simulink model "WiperCtrl"  (R2023b)
settings: Solver=FixedStepDiscrete  StartTime=0.0  StopTime=4  FixedStep=5e-5  RelTol=1e-3  EnableMultiTasking=on
values from neighbouring files (symbols this model uses):
  MC_Hardware_Motor_Mechinal_Fric = 0    [ModelParamSet.m]
  MC_Hardware_Motor_Mechinal_Inertia = 1.03e-2    (= 0.0103)    [ModelParamSet.m]
  MC_Hardware_Motor_Mechinal_TF = 8.59e-2    (= 0.0859)    [ModelParamSet.m]
  MC_Hardware_Motor_Rotor_BEMFCoff = 4.294    [ModelParamSet.m]
  MC_Hardware_Motor_Rotor_Pn = 4    [ModelParamSet.m]
  MC_Hardware_Motor_Stator_Ld = 5.6345e-5    (= 5.6345e-05)    [ModelParamSet.m]
  MC_Hardware_Motor_Stator_Lq = 5.6345e-5    (= 5.6345e-05)    [ModelParamSet.m]
  MC_Hardware_Motor_Stator_Rs = 2.86e-2    (= 0.0286)    [ModelParamSet.m]
  MC_Hardware_Power_DC = 13.5    [ModelParamSet.m]
  MC_Hardware_Sample_CurrentNoise = 1e-15    [ModelParamSet.m]
  MC_Hardware_Sample_Rs = 1e-3    (= 0.001)    [ModelParamSet.m]
  MC_Hardware_Sample_VbusNoise = 1e-15    [ModelParamSet.m]
  MC_Sim_BaseStep = 5e-8    (= 5e-08)    [ModelParamSet.m]
  MC_Sim_HighFrequenceStep = 5e-5    (= 5e-05)    [ModelParamSet.m]
  MC_SVPWM_DutyMax = 0.98    [ModelParamSet.m]
  MC_SVPWM_DutyMin = 0.02    [ModelParamSet.m]
libraries: simulink x12, spsVoltageMeasurementLib x2, spsDCVoltageSourceLib x1, spsGroundLib x1, spsPermanentMagnetSynchronousMachineLib x1, spsSeriesRLCBranchLib x1, spsThreePhaseVIMeasurementLib x1, spsUniversalBridgeLib x1, spspowerguiLib x1
(part 1 of 2)
settings Model: SimulationMode=accelerator  Creator=YXuan  LastModifiedBy=YXuan
settings SolverCC: AllowMultiTaskInputOutput=on  PositivePriorityOrder=on  AutoInsertRateTranBlk=on
settings OptimizationCC: DefaultParameterBehavior=Inlined  EnhancedBackFolding=on  PassReuseOutputArgsAs=Individual arguments  ZeroExternalMemoryAtStartup=off  ZeroInternalMemoryAtStartup=off  OptimizeBlockOrder=speed  DifferentSizesBufferReuse=on  OptimizationCustomize=off  EfficientTunableParamExpr=on
settings DebuggingCC: ParameterPrecisionLossMsg=none  ParameterTunabilityLossMsg=error
settings SFSimCC: MATLABDynamicMemAlloc=off
settings RTWCC: Description=Embedded Coder  SystemTargetFile=ert.tlc  GenCodeOnly=on  TemplateMakefile=ert_default_tmf  Toolchain=Microsoft Visual C++ 2022 v17.0 | nmake (64-bit Windows)
settings CodeAppCC: ForceParamTrailComments=on  IgnoreCustomStorageClasses=off  OperatorAnnotations=on  SimulinkDataObjDesc=on  SFDataObjDesc=on  InsertBlockDesc=on
settings ERTTargetCC: TargetLangStandard=C99 (ISO)  GenerateSampleERTMain=on  InlinedParameterPlacement=NonHierarchical  ERTCustomFileTemplate=example_file_process.tlc

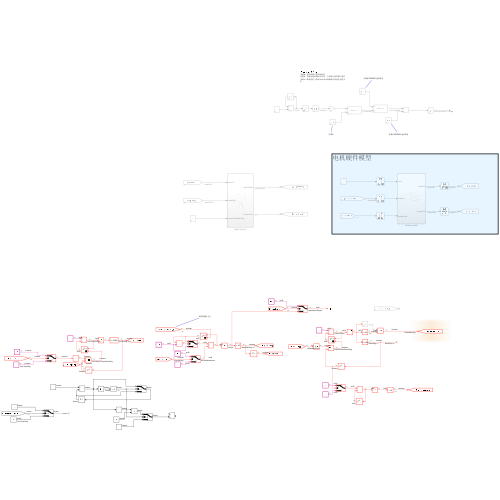
[thumbnail: Simulink's stored preview of the top-level diagram]
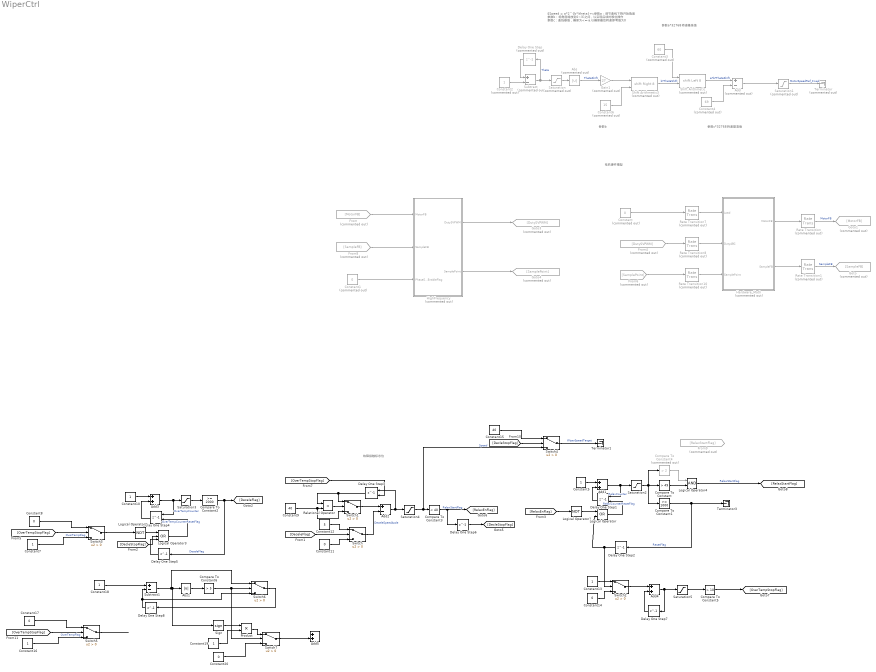
== system WiperCtrl ==
  note: 故障接触标志位
  note: $Speed = a*2^{b*\theta}+c$
      | 参数a：调节曲线下降开始角度
      | 参数b：将角度缩放到0~31之间，以实现后续的移位操作
      | 参数c：曲线基值，确保为<=-a,以确保最后转速参考值为0
  note: 参数a*32768/转速基准值
  note: 电机硬件模型
  note: 参数c*32768/转速基准值
  note: 参数b
  Abs : Abs  Commented=on  SaturateOnIntegerOverflow=off
  Abs1 : Abs  SaturateOnIntegerOverflow=off
  Add : Sum  Commented=on  Inputs=+-
  Add{1,3..5} (4 alike) : Sum
  Add2 : Sum  Inputs=+-
  Compare To Constant : simulink/Logic and Bit Operations/Compare To Constant  relop=>  const=49  OutDataTypeStr=boolean
  Compare To Constant1 : simulink/Logic and Bit Operations/Compare To Constant  relop=>=  const=1000  OutDataTypeStr=boolean
  Compare To Constant2 : simulink/Logic and Bit Operations/Compare To Constant  relop=>=  const=2000  OutDataTypeStr=boolean
  Compare To Constant3 : simulink/Logic and Bit Operations/Compare To Constant  relop=<  const=40  OutDataTypeStr=boolean
  Compare To Constant4 : simulink/Logic and Bit Operations/Compare To Constant  Commented=on  relop=>  const=2  OutDataTypeStr=boolean
  Compare To Constant5 : simulink/Logic and Bit Operations/Compare To Constant  relop=>  const=10  OutDataTypeStr=boolean
  Compare To Constant6 : simulink/Logic and Bit Operations/Compare To Constant  relop=>  const=5  OutDataTypeStr=boolean
  Constant : Constant  Commented=on  Value=0
  Constant1 : Constant  Commented=on  Value=0  OutDataTypeStr=boolean
  Constant{5,10,13,18..19} (5 alike) : Constant  OutDataTypeStr=int32
  Constant11 : Constant  Value=0  OutDataTypeStr=int32
  Constant12 : Constant  Value=5  OutDataTypeStr=int32
  Constant14 : Constant  Value=0  OutDataTypeStr=int32
  Constant15 : Constant  Value=40  OutDataTypeStr=int32
  Constant16 : Constant  OutDataTypeStr=boolean
  Constant17 : Constant  Value=0  OutDataTypeStr=boolean
  Constant2 : Constant  Commented=on  OutDataTypeStr=int32
  Constant20 : Constant  Value=0  OutDataTypeStr=int32
  Constant3 : Constant  Commented=on  Value=60  OutDataTypeStr=int32
  Constant4 : Constant  Commented=on  Value=69  OutDataTypeStr=int16
  Constant6 : Constant  Commented=on  Value=15  OutDataTypeStr=int16
  Constant7 : Constant  OutDataTypeStr=boolean
  Constant8 : Constant  Value=0  OutDataTypeStr=boolean
  Constant9 : Constant  Value=40  OutDataTypeStr=int32
  Delay One Step : Delay  Commented=on  DelayLength=1  InitialCondition=int32(32768)
  Delay One Step1 : Delay  DelayLength=1  InitialCondition=int32(0)  ExternalReset=Level
      settings: InputPortMap=u0,r5
  Delay One Step2 : Delay  DelayLength=1  InitialCondition=boolean(0)
  Delay One Step3 : Delay  DelayLength=1  InitialCondition=60  ExternalReset=Level
      settings: InputPortMap=u0,r5
  Delay One Step4 : Delay  DelayLength=1  InitialCondition=int32(0)  ExternalReset=Level
      settings: InputPortMap=u0,r5
  Delay One Step5 : Delay  DelayLength=1  InitialCondition=boolean(0)
  Delay One Step6 : Delay  DelayLength=1  InitialCondition=boolean(0)
  Delay One Step7 : Delay  DelayLength=1  InitialCondition=int32(0)
  Delay One Step8 : Delay  DelayLength=1
  From : From  Commented=on  GotoTag=MotorFB
  From4 : From  Commented=on  GotoTag=DutySVPWM
  From6 : From  Commented=on  GotoTag=SamplePoint
  From8 : From  Commented=on  GotoTag=SampleFB
  From9 : From  Commented=on  GotoTag=RelaxStartFlag
  Gain1 : Gain  Commented=on  Gain=27  ParamDataTypeStr=int16  OutDataTypeStr=int32  RndMeth=Simplest
  Goto : Goto  Commented=on  GotoTag=SampleFB
  Goto1 : Goto  Commented=on  GotoTag=MotorFB
  Goto3 : Goto  Commented=on  GotoTag=DutySVPWM
  Goto4 : Goto  Commented=on  GotoTag=SamplePoint
  Hardware_Math : Subsystem  Commented=on  SystemSampleTime=MC_Sim_BaseStep  VariantControl=MC_Hardware_Motor_Model ==1&MC_Hardware_MotorMOS_Model==1
  HighFrequency : Subsystem  Commented=on
  Logical Operator : Logic  Operator=OR  AllPortsSameDT=off  OutDataTypeStr=boolean
  Logical Operator1 : Logic  Operator=NOT  AllPortsSameDT=off  OutDataTypeStr=boolean
  Logical Operator2 : Logic  Operator=NOT  AllPortsSameDT=off  OutDataTypeStr=boolean
  Logical Operator3 : Logic  Operator=OR  Inputs=3  AllPortsSameDT=off  OutDataTypeStr=boolean
  Logical Operator4 : Logic  AllPortsSameDT=off  OutDataTypeStr=boolean
  Product : Product
  Rate Transition : RateTransition  Commented=on  OutPortSampleTime=MC_Sim_HighFrequenceStep
  Rate Transition1 : RateTransition  Commented=on  OutPortSampleTime=MC_Sim_HighFrequenceStep
  Rate Transition10 : RateTransition  Commented=on  OutPortSampleTime=MC_Sim_BaseStep
  Rate Transition7 : RateTransition  Commented=on  OutPortSampleTime=MC_Sim_BaseStep
  Rate Transition8 : RateTransition  Commented=on  OutPortSampleTime=MC_Sim_BaseStep
  Relational Operator : RelationalOperator  Operator=<  OutDataTypeStr=boolean  RndMeth=Simplest  InputSameDT=off
  Saturation : Saturate  Commented=on  UpperLimit=32768  LowerLimit=-32768  OutDataTypeStr=int32  RndMeth=Simplest
  Saturation1 : Saturate  Commented=on  UpperLimit=4800  LowerLimit=0
  Saturation2 : Saturate  UpperLimit=1500  LowerLimit=-1
  Saturation3 : Saturate  UpperLimit=2001  LowerLimit=-1
  Saturation4 : Saturate  UpperLimit=60  LowerLimit=30  OutDataTypeStr=int32  RndMeth=Simplest
  Saturation5 : Saturate  UpperLimit=20  LowerLimit=-1
  Shift Arithmetic : ArithShift  Commented=on  BitShiftNumberSource=Input port  BitShiftNumber=8  BitShiftDirection=Left
      settings: InputPortMap=u0,p1
  Shift Arithmetic3 : ArithShift  Commented=on  BitShiftNumberSource=Input port  BitShiftNumber=8  BitShiftDirection=Right
      settings: InputPortMap=u0,p1
  Sign : Signum
  Subtract : Sum  Commented=on  Inputs=+-
  Subtract1 : Sum  Inputs=+-
  Switch{,1..7} (8 alike) : Switch  Criteria=u2 > Threshold  SaturateOnIntegerOverflow=off  InputSameDT=off
  Terminator : Terminator  Commented=on
  Terminator1 : Terminator
  Terminator3 : Terminator
  wires:
  Hardware_Math/2(SampleFB) -> Rate Transition1/1
  Rate Transition8/1 -> Hardware_Math/2(DutyABC)
  Hardware_Math/1(MotorFB) -> Rate Transition/1
  From6/1 -> Rate Transition10/1
  From4/1 -> Rate Transition8/1
  Rate Transition1/1 -> Goto/1  "SampleFB"
  Constant/1 -> Rate Transition7/1
  Rate Transition10/1 -> Hardware_Math/3(SamplePoint)
  Rate Transition7/1 -> Hardware_Math/1(Load)
  Rate Transition/1 -> Goto1/1  "MotorFB"
  From8/1 -> HighFrequency/2(SampleFB)
  From/1 -> HighFrequency/1(MotorFB)
  Constant1/1 -> HighFrequency/3(PhaseShortEnableFlag)
  HighFrequency/2(SamplePoint) -> Goto4/1
  HighFrequency/1(DutySVPWM) -> Goto3/1
  Subtract/1 -> Saturation/1, Delay One Step/1  "Theta"
  Delay One Step/1 -> Subtract/1
  Constant2/1 -> Subtract/2
  Saturation/1 -> Abs/1
  Abs/1 -> Gain1/1  "ThetaShift"
  Constant3/1 -> Shift Arithmetic/1
  Shift Arithmetic/1 -> Add/1  "a*b*ThetaShift"
  Constant4/1 -> Add/2
  Shift Arithmetic3/1 -> Shift Arithmetic/2  "b*ThetaShift"
  Gain1/1 -> Shift Arithmetic3/1
  Constant6/1 -> Shift Arithmetic3/2
  Add/1 -> Saturation1/1
  Saturation1/1 -> Terminator/1  "MotorSpeedRef_Fixed"
  Constant5/1 -> Add1/1
  Add1/1 -> Saturation2/1, Delay One Step1/1  "RelaxCounter"
  Delay One Step1/1 -> Add1/2
  Saturation2/1 -> Compare To Constant/1, Compare To Constant4/1, Compare To Constant1/1
  Logical Operator4/1 -> [RelaxStartFlag]  "RelaxStartFlag"
  Compare To Constant1/1 -> Terminator3/1, Delay One Step2/1  "ResetFlag"
  Delay One Step2/1 -> Logical Operator/2, Switch2/2
  Logical Operator/1 -> Delay One Step1/2  "RelaxCounterResetFlag"
  Logical Operator1/1 -> Logical Operator/1
  Constant10/1 -> Add3/1
  Add3/1 -> Saturation3/1, Delay One Step4/1  "OverTempCounter"
  Delay One Step4/1 -> Add3/2
  Switch3/1 -> Logical Operator2/1
  Saturation3/1 -> Compare To Constant2/1
  Compare To Constant2/1 -> [DeceleFlag], Delay One Step5/1  "DeceleFlag"
  Logical Operator2/1 -> Logical Operator3/1
  Logical Operator3/1 -> Delay One Step4/2  "OverTempCounterResetFlag"
  Delay One Step5/1 -> Logical Operator3/3
  [DeceleFlag] -> Switch/2
  Constant11/1 -> Switch/3
  Constant12/1 -> Switch/1
  Switch/1 -> Add2/2  "DeceleSpeedAccle"
  Switch1/1 -> Add2/1
  Delay One Step3/1 -> Switch1/1, Relational Operator/1
  Constant9/1 -> Relational Operator/2, Switch1/3
  Relational Operator/1 -> Switch1/2
  Add2/1 -> Saturation4/1, Delay One Step3/1
  Saturation4/1 -> Switch4/3, Compare To Constant3/1  "Speed"
  Compare To Constant3/1 -> [RelaxEnFlag], Delay One Step6/1  "RelaxStartFlag"
  Compare To Constant4/1 -> Logical Operator4/1
  Compare To Constant/1 -> Logical Operator4/2
  [DecleStopFlag] -> Logical Operator3/2
  Delay One Step6/1 -> [DecleStopFlag]
  [RelaxEnFlag] -> Logical Operator1/1
  Constant13/1 -> Switch2/1
  Constant14/1 -> Switch2/3
  Switch2/1 -> Add4/1
  Add4/1 -> Saturation5/1, Delay One Step7/1
  Delay One Step7/1 -> Add4/2
  Saturation5/1 -> Compare To Constant5/1
  Compare To Constant5/1 -> [OverTempStopFlag]
  [OverTempStopFlag] -> Switch3/2
  Constant7/1 -> Switch3/3  "OverTempFlag"
  Constant8/1 -> Switch3/1
  [OverTempStopFlag] -> Delay One Step3/2
  [DecleStopFlag] -> Switch4/2
  Constant15/1 -> Switch4/1
  Switch4/1 -> Terminator1/1  "WiperSpeedTarget"
  Constant17/1 -> Switch5/1
  Constant16/1 -> Switch5/3  "OverTempFlag"
  [OverTempStopFlag] -> Switch5/2
  Switch5/1 -> ?
  Constant18/1 -> Subtract1/1
  Subtract1/1 -> Switch6/1, Sign/1, Abs1/1
  Delay One Step8/1 -> Subtract1/2, Switch6/3
  Compare To Constant6/1 -> Switch7/2, Switch6/2
  Switch6/1 -> Delay One Step8/1
  Abs1/1 -> Compare To Constant6/1
  Sign/1 -> Product/1
  Constant19/1 -> Product/2
  Product/1 -> Switch7/1
  Constant20/1 -> Switch7/3
  Switch7/1 -> Add5/2

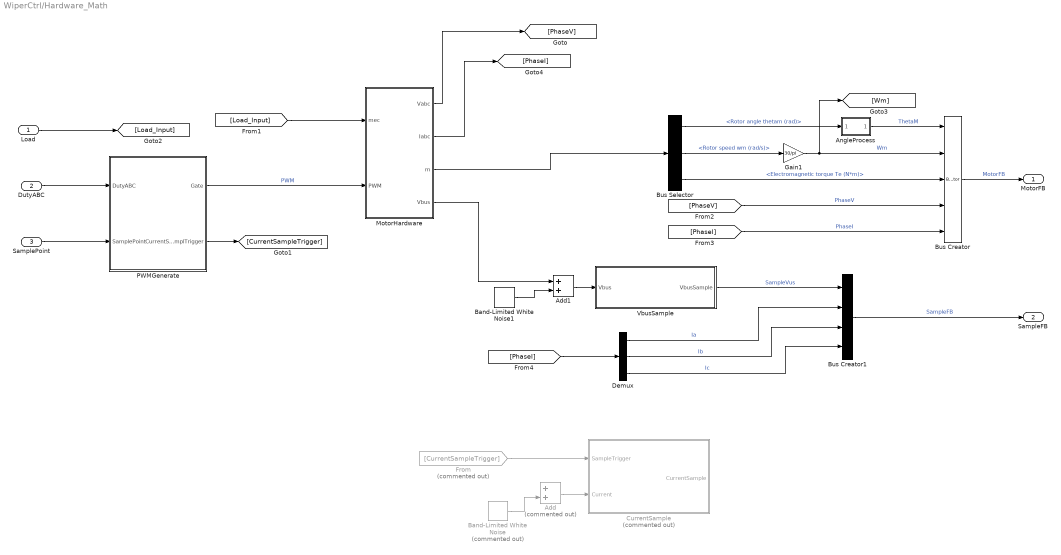
== system WiperCtrl/Hardware_Math ==
  Load : Inport
  DutyABC : Inport  Port=2
  SamplePoint : Inport  Port=3
  Add : Sum  Commented=on
  Add1 : Sum
  AngleProcess : Subsystem
  Band-Limited White Noise : simulink/Sources/Band-Limited White Noise  Commented=on  Cov=[MC_Hardware_Sample_CurrentNoise]  Ts=MC_Sim_BaseStep  seed=[23341]
  Band-Limited White Noise1 : simulink/Sources/Band-Limited White Noise  Cov=[MC_Hardware_Sample_VbusNoise]  Ts=MC_Sim_BaseStep  seed=[23341]
  Bus Creator : BusCreator  Inputs=5
  Bus Creator1 : BusCreator  Inputs=4
  Bus Selector : BusSelector  OutputSignals=Rotor angle thetam (rad),Rotor speed wm (rad/s),Electromagnetic torque Te (N*m)
  CurrentSample : Subsystem  Commented=on  Variant=on  VariantControlMode=label  VariantControl=CurrentSample  LabelModeActiveChoice=CurrentSample
  Demux : Demux  Outputs=3
  From : From  Commented=on  GotoTag=CurrentSampleTrigger
  Gain1 : Gain  Gain=30/pi
  MotorHardware : Subsystem
  PWMGenerate : Subsystem  SystemSampleTime=MC_Sim_BaseStep
  VbusSample : Subsystem
  MotorFB : Outport
  SampleFB : Outport  Port=2
  wires:
  Band-Limited White Noise/1 -> Add/2
  Add/1 -> CurrentSample/2(Current)
  Add1/1 -> VbusSample/1(Vbus)
  Band-Limited White Noise1/1 -> Add1/2
  From/1 -> CurrentSample/1(SampleTrigger)
  PWMGenerate/2(CurrentSamplTrigger) -> [CurrentSampleTrigger]
  Bus Selector/2 -> Gain1/1  "<Rotor speed wm (rad/s)>"
  DutyABC/1 -> PWMGenerate/1(DutyABC)
  Bus Selector/1 -> AngleProcess/1(In1)  "<Rotor angle thetam (rad)>"
  SamplePoint/1 -> PWMGenerate/2(SamplePoint)
  Bus Selector/3 -> Bus Creator/3  "<Electromagnetic torque Te (N*m)>"
  Load/1 -> [Load_Input]
  Gain1/1 -> [Wm], Bus Creator/2  "Wm"
  AngleProcess/1(Out1) -> Bus Creator/1  "ThetaM"
  [PhaseV] -> Bus Creator/4  "PhaseV"
  [PhaseI] -> Bus Creator/5  "PhaseI"
  Bus Creator/1 -> MotorFB/1  "MotorFB"
  VbusSample/1(VbusSample) -> Bus Creator1/1  "SampleVus"
  Bus Creator1/1 -> SampleFB/1  "SampleFB"
  [Load_Input] -> MotorHardware/1(mec)
  PWMGenerate/1(Gate) -> MotorHardware/2(PWM)  "PWM"
  MotorHardware/1(Vabc) -> [PhaseV]
  MotorHardware/2(Iabc) -> [PhaseI]
  MotorHardware/3(m) -> Bus Selector/1
  MotorHardware/4(Vbus) -> Add1/1
  Demux/1 -> Bus Creator1/2  "Ia"
  Demux/2 -> Bus Creator1/3  "Ib"
  Demux/3 -> Bus Creator1/4  "Ic"
  [PhaseI] -> Demux/1

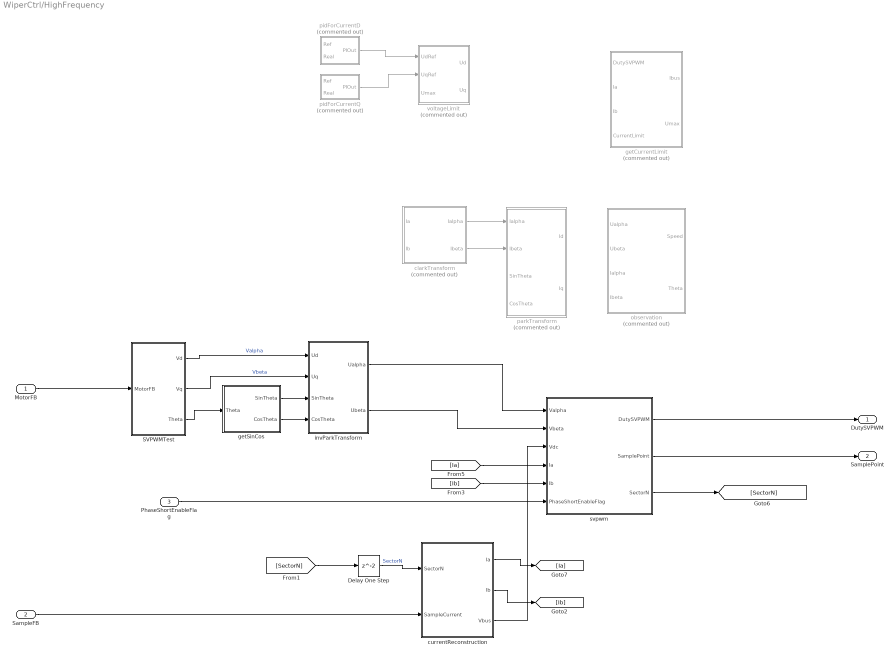
== system WiperCtrl/HighFrequency ==
  MotorFB : Inport
  SampleFB : Inport  Port=2
  PhaseShortEnableFlag : Inport  Port=3
  Delay One Step : Delay
  SVPWMTest : Subsystem
  clarkTransform : Subsystem  Commented=on
  currentReconstruction : Subsystem
  getCurrentLimit : Subsystem  Commented=on
  getSinCos : Subsystem
  invParkTransform : Subsystem
  observation : Subsystem  Commented=on  Variant=on  VariantControlMode=label  VariantControl=observation  LabelModeActiveChoice=observation
  parkTransform : Subsystem  Commented=on
  pidForCurrentD : Subsystem  Commented=on
  pidForCurrentQ : Subsystem  Commented=on
  svpwm : Subsystem  TreatAsAtomicUnit=on  SystemSampleTime=MC_Sim_HighFrequenceStep
  voltageLimit : Subsystem  Commented=on
  DutySVPWM : Outport
  SamplePoint : Outport  Port=2
  wires:
  [SectorN] -> Delay One Step/1
  PhaseShortEnableFlag/1 -> svpwm/6(PhaseShortEnableFlag)
  svpwm/3(SectorN) -> [SectorN]
  [Ia] -> svpwm/4(Ia)
  [Ib] -> svpwm/5(Ib)
  currentReconstruction/2(Ib) -> [Ib]
  currentReconstruction/1(Ia) -> [Ia]
  Delay One Step/1 -> currentReconstruction/1(SectorN)  "SectorN"
  svpwm/2(SamplePoint) -> SamplePoint/1
  svpwm/1(DutySVPWM) -> DutySVPWM/1
  SampleFB/1 -> currentReconstruction/2(SampleCurrent)
  pidForCurrentD/1(PIOut) -> voltageLimit/1(UdRef)
  pidForCurrentQ/1(PIOut) -> voltageLimit/2(UqRef)
  clarkTransform/1(Ialpha) -> parkTransform/1(Ialpha)
  clarkTransform/2(Ibeta) -> parkTransform/2(Ibeta)
  getSinCos/1(SinTheta) -> invParkTransform/3(SinTheta)
  getSinCos/2(CosTheta) -> invParkTransform/4(CosTheta)
  SVPWMTest/3(Theta) -> getSinCos/1(Theta)
  SVPWMTest/1(Vd) -> invParkTransform/1(Ud)  "Valpha"
  SVPWMTest/2(Vq) -> invParkTransform/2(Uq)  "Vbeta"
  invParkTransform/2(Ubeta) -> svpwm/2(Vbeta)
  invParkTransform/1(Ualpha) -> svpwm/1(Valpha)
  MotorFB/1 -> SVPWMTest/1(MotorFB)
  currentReconstruction/3(Vbus) -> svpwm/3(Vdc)

== system WiperCtrl/Hardware_Math/AngleProcess ==
  In1 : Inport
  Constant : Constant  Value=2*pi  SampleTime=-1
  Mod : Math  Operator=mod
  Out1 : Outport
  wires:
  Mod/1 -> Out1/1
  In1/1 -> Mod/1
  Constant/1 -> Mod/2

== system WiperCtrl/Hardware_Math/CurrentSample ==
  SampleTrigger : Inport
  Current : Inport  Port=2
  "CurrentSample(OneRS) " : Subsystem  VariantControl=CurrentSample
  CurrentSample : Outport

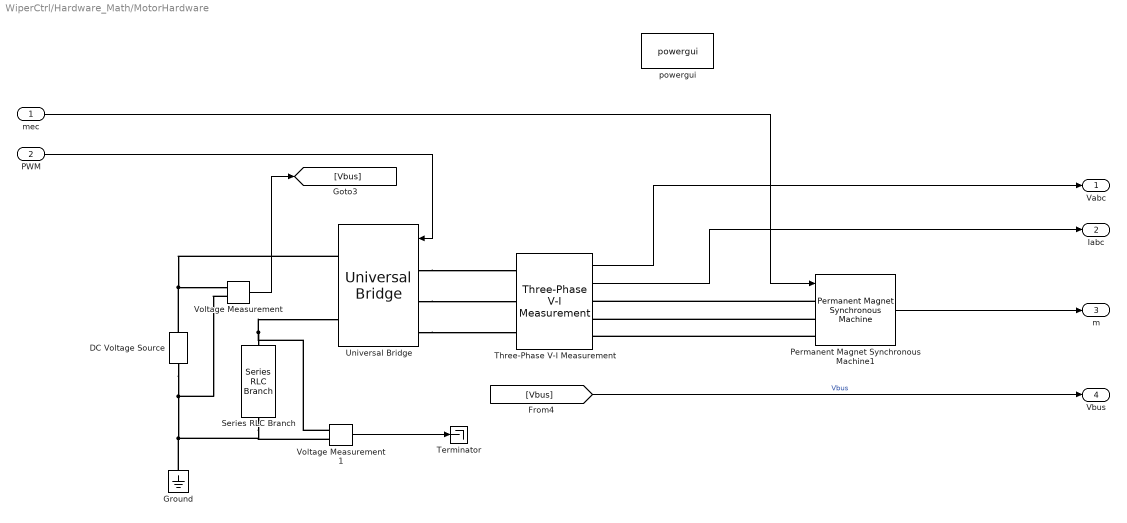
== system WiperCtrl/Hardware_Math/MotorHardware ==
  mec : Inport
  PWM : Inport  Port=2
  DC Voltage Source : spsDCVoltageSourceLib/DC Voltage Source  Amplitude=MC_Hardware_Power_DC  Measurements=None
  Ground : spsGroundLib/Ground  LConnTagsString=a
  Permanent Magnet Synchronous Machine1 : spsPermanentMagnetSynchronousMachineLib/Permanent Magnet Synchronous Machine  NbPhases=3  FluxDistribution=Sinusoidal  RotorType=Salient-pole  MechanicalLoad=Torque Tm  PresetModel=No  ShowDetailedParameters=on  MeasurementBus=off  Resistance=double(MC_Hardware_Motor_Stator_Rs)  Inductance=8.5e-3  dqInductances=[double(MC_Hardware_Motor_Stator_Ld),double(MC_Hardware_Motor_Stator_Lq)]  La=0.000395  MachineConstant=Voltage Constant (V_peak L-L / krpm)  Flux=0.0059185  VoltageCst=double(MC_Hardware_Motor_Rotor_BEMFCoff)  TorqueCst=0.035511  Flat=120  Mechanical=[double(MC_Hardware_Motor_Mechinal_Inertia) double(MC_Hardware_Motor_Mechinal_Fric) double(MC_Hardware_Motor_Rotor_Pn) double(MC_Hardware_Motor_Mechinal_TF)]  PolePairs=4  InitialConditions=[0,0, 0,0]  InitialConditions5ph=[0 0 0 0 0 0]  RefAngle=Aligned with phase A axis (original Park)  IterativeDiscreteModel=Trapezoidal non iterative  TsBlock=-1  TsPowergui=0
  Series RLC Branch : spsSeriesRLCBranchLib/Series RLC Branch  LConnTagsString=__new0  RConnTagsString=__new0  BranchType=R  Resistance=MC_Hardware_Sample_Rs  Inductance=1e-3  SetiL0=off  InitialCurrent=0  Capacitance=1e-6  Setx0=off  InitialVoltage=0  Measurements=None
  Terminator : Terminator
  Three-Phase V-I Measurement : spsThreePhaseVIMeasurementLib/Three-Phase V-I Measurement  VoltageMeasurement=phase-to-ground  SetLabelV=off  LabelV=Vabc  Vpu=off  VpuLL=off  CurrentMeasurement=yes  SetLabelI=off  LabelI=Iabc  Ipu=off  Pbase=100e6  Vbase=500e3  OutputType=Complex  PhasorSimulation=off  PSBequivalent=0
  Universal Bridge : spsUniversalBridgeLib/Universal Bridge  Arms=3  SnubberResistance=1e5  SnubberCapacitance=inf  Device=MOSFET / Diodes  Ron=MC_Hardware_MOS_Rds  Lon=0  ForwardVoltages="[  0  0  ]"  ForwardVoltage=MC_Hardware_MOS_Threshold  GTOparameters=[ 10e-6 , 20e-6 ]  IGBTparameters=[ 1e-6 , 2e-6 ]  Measurements=None  Measurements_2=None  converterType=Rectifier
  Voltage Measurement : spsVoltageMeasurementLib/Voltage Measurement  PhasorSimulation=off  OutputType=Complex  PSBequivalent=0
  Voltage Measurement1 : spsVoltageMeasurementLib/Voltage Measurement  PhasorSimulation=off  OutputType=Complex  PSBequivalent=0
  powergui : spspowerguiLib/powergui  Priority=1  SimulationMode=Discrete  SampleTime=MC_Sim_BaseStep  frequency=60  Iterations=50  frequencyindice=0  Pbase=100e6  ErrMax=1e-4  UnitsV=kV  UnitsW=MW  buscounter=0  FunctionMessages=off  echomessages=off  EnableUseOfTLC=off  CurrentSourceSwitches=off  DisableSnubberDevices=off  DisableRonSwitches=off  DisableVfSwitches=off  DisplayEquations=off  AutomaticDiscreteSolvers=off  SolverType=Tustin/Backward Euler (TBE)  Interpol=off  ExternalGateDelay=off  methode=off  Ts=100  x0status=blocks  SPID=on  SwTol=0  HookPort=off  NonlinearTolerance=1e-4  nMaxIteration=100  ContinueOnMaxIteration=off  RestoreLinks=warning  ResistiveCurrentMeasurement=off  Frange=[0:2:500]  Ylog=off  Xlog=on  ShowGrid=off  save=off  variable=ZData  structure=0  ZoomFFT=off  StartTime=0.0  cycles=1  DisplayStyle=1  fundamental=60  FreqAxis=off  MaxFrequency=1000  frequencyindicesteady=1  RmsSteady=1  display=off
  Vabc : Outport
  Iabc : Outport  Port=2
  m : Outport  Port=3
  Vbus : Outport  Port=4
  wires:
  mec/1 -> Permanent Magnet Synchronous Machine1/1
  [Vbus] -> Vbus/1  "Vbus"
  Voltage Measurement/1 -> [Vbus]
  Three-Phase V-I Measurement/1 -> Vabc/1
  Three-Phase V-I Measurement/2 -> Iabc/1
  PWM/1 -> Universal Bridge/1
  Permanent Magnet Synchronous Machine1/1 -> m/1
  Voltage Measurement1/1 -> Terminator/1
  connections:
  Permanent Magnet Synchronous Machine1/LConn2 -- Three-Phase V-I Measurement/RConn2
  DC Voltage Source/RConn1 -- Universal Bridge/RConn1 -- Voltage Measurement/LConn1
  Voltage Measurement/LConn2 -- Voltage Measurement1/LConn2 -- Series RLC Branch/RConn1 -- Ground/LConn1 -- DC Voltage Source/LConn1
  Permanent Magnet Synchronous Machine1/LConn1 -- Three-Phase V-I Measurement/RConn1
  Permanent Magnet Synchronous Machine1/LConn3 -- Three-Phase V-I Measurement/RConn3
  Universal Bridge/LConn1 -- Three-Phase V-I Measurement/LConn1
  Universal Bridge/LConn2 -- Three-Phase V-I Measurement/LConn2
  Universal Bridge/LConn3 -- Three-Phase V-I Measurement/LConn3
  Voltage Measurement1/LConn1 -- Series RLC Branch/LConn1 -- Universal Bridge/RConn2

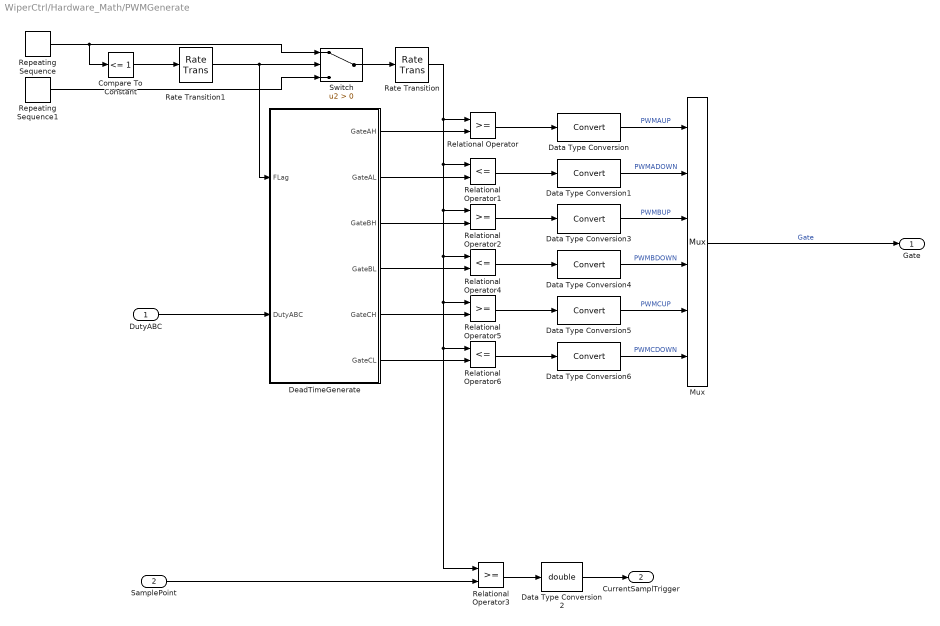
== system WiperCtrl/Hardware_Math/PWMGenerate ==
  DutyABC : Inport
  SamplePoint : Inport  Port=2
  Compare To Constant : simulink/Logic and Bit Operations/Compare To Constant  relop=<=  const=1  OutDataTypeStr=boolean
  Data Type Conversion{,1,3..6} (6 alike) : DataTypeConversion  SaturateOnIntegerOverflow=off  RndMeth=Floor
  Data Type Conversion2 : DataTypeConversion  OutDataTypeStr=double  SaturateOnIntegerOverflow=off  RndMeth=Floor
  DeadTimeGenerate : Subsystem
  Mux : Mux  Inputs=6
  Rate Transition : RateTransition  OutPortSampleTime=MC_Sim_BaseStep
  Rate Transition1 : RateTransition  OutPortSampleTime=MC_Sim_BaseStep
  Relational Operator{,2..3,5} (4 alike) : RelationalOperator  OutDataTypeStr=boolean  RndMeth=Simplest  InputSameDT=off
  Relational Operator1 : RelationalOperator  Operator=<=  OutDataTypeStr=boolean  RndMeth=Simplest  InputSameDT=off
  Relational Operator4 : RelationalOperator  Operator=<=  OutDataTypeStr=boolean  RndMeth=Simplest  InputSameDT=off
  Relational Operator6 : RelationalOperator  Operator=<=  OutDataTypeStr=boolean  RndMeth=Simplest  InputSameDT=off
  Repeating Sequence : simulink/Sources/Repeating Sequence  rep_seq_t=[0 MC_Sim_HighFrequenceStep/2 MC_Sim_HighFrequenceStep]  rep_seq_y=[0 1 2]
  Repeating Sequence1 : simulink/Sources/Repeating Sequence  rep_seq_t=[0 MC_Sim_HighFrequenceStep/2 MC_Sim_HighFrequenceStep]  rep_seq_y=[2 1 0]
  Switch : Switch  Criteria=u2 > Threshold  SaturateOnIntegerOverflow=off  InputSameDT=off
  Gate : Outport
  CurrentSamplTrigger : Outport  Port=2
  wires:
  Data Type Conversion6/1 -> Mux/6  "PWMCDOWN"
  Data Type Conversion5/1 -> Mux/5  "PWMCUP"
  Data Type Conversion4/1 -> Mux/4  "PWMBDOWN"
  Data Type Conversion3/1 -> Mux/3  "PWMBUP"
  Data Type Conversion1/1 -> Mux/2  "PWMADOWN"
  Data Type Conversion/1 -> Mux/1  "PWMAUP"
  DeadTimeGenerate/6(GateCL) -> Relational Operator6/2
  DeadTimeGenerate/5(GateCH) -> Relational Operator5/2
  DeadTimeGenerate/4(GateBL) -> Relational Operator4/2
  DeadTimeGenerate/3(GateBH) -> Relational Operator2/2
  Relational Operator6/1 -> Data Type Conversion6/1
  Relational Operator5/1 -> Data Type Conversion5/1
  Relational Operator4/1 -> Data Type Conversion4/1
  Relational Operator2/1 -> Data Type Conversion3/1
  Relational Operator1/1 -> Data Type Conversion1/1
  Relational Operator/1 -> Data Type Conversion/1
  Repeating Sequence/1 -> Switch/1, Compare To Constant/1
  Repeating Sequence1/1 -> Switch/3
  DutyABC/1 -> DeadTimeGenerate/2(DutyABC)
  DeadTimeGenerate/1(GateAH) -> Relational Operator/2
  Switch/1 -> Rate Transition/1
  DeadTimeGenerate/2(GateAL) -> Relational Operator1/2
  Relational Operator3/1 -> Data Type Conversion2/1
  SamplePoint/1 -> Relational Operator3/2
  Data Type Conversion2/1 -> CurrentSamplTrigger/1
  Compare To Constant/1 -> Rate Transition1/1
  Mux/1 -> Gate/1  "Gate"
  Rate Transition/1 -> Relational Operator/1, Relational Operator1/1, Relational Operator3/1, Relational Operator6/1, Relational Operator5/1, Relational Operator4/1, Relational Operator2/1
  Rate Transition1/1 -> DeadTimeGenerate/1(FLag), Switch/2

== system WiperCtrl/Hardware_Math/VbusSample ==
  Vbus : Inport
  ADCOffset : Constant  Value=0  SampleTime=-1
  ADCQuality : Gain
  Add : Sum
  VbusSample : Outport
  wires:
  Vbus/1 -> Add/2
  Add/1 -> ADCQuality/1
  ADCQuality/1 -> VbusSample/1
  ADCOffset/1 -> Add/1

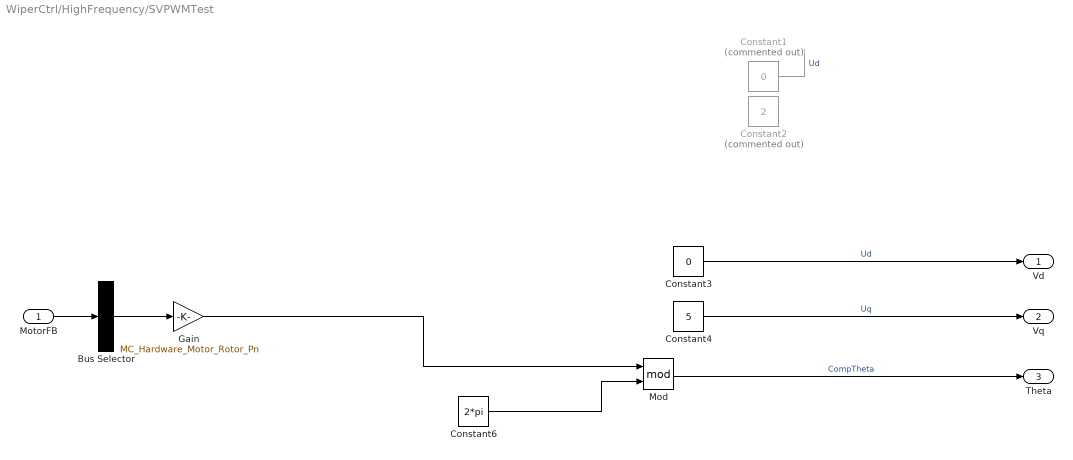
== system WiperCtrl/HighFrequency/SVPWMTest ==
  MotorFB : Inport
  Bus Selector : BusSelector  OutputSignals=ThetaM  OutputAsBus=on
  Constant1 : Constant  Commented=on  Value=0  SampleTime=MC_Sim_HighFrequenceStep
  Constant2 : Constant  Commented=on  Value=2  SampleTime=MC_Sim_HighFrequenceStep
  Constant3 : Constant  Value=0
  Constant4 : Constant  Value=5
  Constant6 : Constant  Value=2*pi
  Gain : Gain  Gain=MC_Hardware_Motor_Rotor_Pn
  Mod : Math  Operator=mod
  Vd : Outport
  Vq : Outport  Port=2
  Theta : Outport  Port=3
  wires:
  Constant3/1 -> Vd/1  "Ud"
  Constant4/1 -> Vq/1  "Uq"
  Constant1/1 -> ?  "Ud"
  Constant6/1 -> Mod/2
  Mod/1 -> Theta/1  "CompTheta"
  MotorFB/1 -> Bus Selector/1
  Bus Selector/1 -> Gain/1
  Gain/1 -> Mod/1

== system WiperCtrl/HighFrequency/clarkTransform ==
  Ia : Inport
  Ib : Inport  Port=2
  a_plus_2b : Sum  Inputs=+++  RndMeth=Simplest  OutDataTypeStr=Inherit: Same as first input
  one_by_sqrt3 : Gain  Gain=1/sqrt(3)  RndMeth=Simplest  OutDataTypeStr=Inherit: Same as input
  Ialpha : Outport
  Ibeta : Outport  Port=2
  wires:
  a_plus_2b/1 -> one_by_sqrt3/1
  Ib/1 -> a_plus_2b/3, a_plus_2b/2
  Ia/1 -> a_plus_2b/1, Ialpha/1
  one_by_sqrt3/1 -> Ibeta/1

== system WiperCtrl/HighFrequency/currentReconstruction ==
  SectorN : Inport
  SampleCurrent : Inport  Port=2
  Bus Selector : BusSelector  OutputSignals=Ia,Ib,SampleVus
  Demux : Demux  Commented=on  Outputs=2
  Terminator : Terminator
  currentPreProcess : Subsystem  Commented=on
  getCurrentPhase : Subsystem  Commented=on
  Ia : Outport
  Ib : Outport  Port=2
  Vbus : Outport  Port=3
  wires:
  SampleCurrent/1 -> Bus Selector/1
  Demux/1 -> currentPreProcess/1(SampleCurrentPoint1)  "SampleCurrentPoint1"
  Demux/2 -> currentPreProcess/2(SampleCurrentPoint2)  "SampleCurrentPoint2"
  currentPreProcess/1(I1) -> getCurrentPhase/2(I1)
  currentPreProcess/2(-I2) -> getCurrentPhase/3(-I2)
  currentPreProcess/3(I2-I1) -> getCurrentPhase/4(I2-I1)
  SectorN/1 -> Terminator/1
  Bus Selector/1 -> Ia/1  "<Ia>"
  Bus Selector/2 -> Ib/1  "<Ib>"
  Bus Selector/3 -> Vbus/1  "<SampleVus>"

== system WiperCtrl/HighFrequency/getCurrentLimit ==
  DutySVPWM : Inport
  Ia : Inport  Port=2
  Ib : Inport  Port=3
  CurrentLimit : Inport  Port=4
  Constant : Constant
  Terminator{,1..3} (4 alike) : Terminator
  Ibus : Outport
  Umax : Outport  Port=2
  wires:
  Constant/1 -> Ibus/1, Umax/1
  Ia/1 -> Terminator1/1
  DutySVPWM/1 -> Terminator/1
  Ib/1 -> Terminator2/1
  CurrentLimit/1 -> Terminator3/1

== system WiperCtrl/HighFrequency/getSinCos ==
  Theta : Inport
  Sin : Trigonometry
  Sin1 : Trigonometry  Operator=cos
  SinTheta : Outport
  CosTheta : Outport  Port=2
  wires:
  Theta/1 -> Sin1/1, Sin/1
  Sin/1 -> SinTheta/1
  Sin1/1 -> CosTheta/1

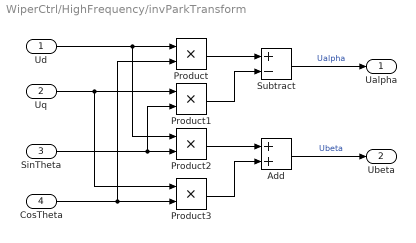
== system WiperCtrl/HighFrequency/invParkTransform ==
  Ud : Inport
  Uq : Inport  Port=2
  SinTheta : Inport  Port=3
  CosTheta : Inport  Port=4
  Add : Sum
  Product{,1..3} (4 alike) : Product
  Subtract : Sum  Inputs=+-
  Ualpha : Outport
  Ubeta : Outport  Port=2
  wires:
  Uq/1 -> Product3/1, Product1/1
  Subtract/1 -> Ualpha/1  "Ualpha"
  CosTheta/1 -> Product/2, Product3/2
  SinTheta/1 -> Product2/2, Product1/2
  Product/1 -> Subtract/1
  Product1/1 -> Subtract/2
  Ud/1 -> Product/1, Product2/1
  Product2/1 -> Add/1
  Product3/1 -> Add/2
  Add/1 -> Ubeta/1  "Ubeta"

== system WiperCtrl/HighFrequency/observation ==
  Ualpha : Inport
  Ubeta : Inport  Port=2
  Ialpha : Inport  Port=3
  Ibeta : Inport  Port=4
  flux : Subsystem  VariantControl=smo1
  longbergur : Subsystem  VariantControl=flux1
  smo : Subsystem  VariantControl=observation
  Speed : Outport
  Theta : Outport  Port=2

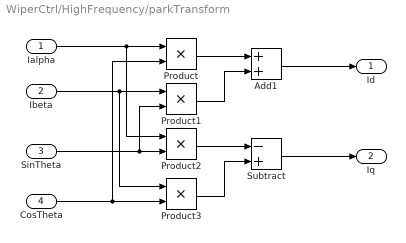
== system WiperCtrl/HighFrequency/parkTransform ==
  Ialpha : Inport
  Ibeta : Inport  Port=2
  SinTheta : Inport  Port=3
  CosTheta : Inport  Port=4
  Add1 : Sum
  Product{,1..3} (4 alike) : Product
  Subtract : Sum  Inputs=-+
  Id : Outport
  Iq : Outport  Port=2
  wires:
  Product3/1 -> Subtract/2
  Product2/1 -> Subtract/1
  Add1/1 -> Id/1
  Subtract/1 -> Iq/1
  Product/1 -> Add1/1
  Product1/1 -> Add1/2
  Ialpha/1 -> Product/1, Product2/1
  Ibeta/1 -> Product3/1, Product1/1
  CosTheta/1 -> Product3/2, Product/2
  SinTheta/1 -> Product2/2, Product1/2

== system WiperCtrl/HighFrequency/pidForCurrentD ==
  Ref : Inport
  Real : Inport  Port=2
  pidConcatenation : Subsystem  Commented=on
  pidPallarConnection : Subsystem
  PIOut : Outport
  wires:
  Ref/1 -> pidPallarConnection/1(Ref)
  Real/1 -> pidPallarConnection/2(Real)
  pidPallarConnection/1(PIOut) -> PIOut/1

== system WiperCtrl/HighFrequency/pidForCurrentQ ==
  Ref : Inport
  Real : Inport  Port=2
  pidConcatenation : Subsystem  Commented=on
  pidPallarConnection : Subsystem
  PIOut : Outport
  wires:
  Ref/1 -> pidPallarConnection/1(Ref)
  Real/1 -> pidPallarConnection/2(Real)
  pidPallarConnection/1(PIOut) -> PIOut/1

== system WiperCtrl/HighFrequency/svpwm ==
  Valpha : Inport
  Vbeta : Inport  Port=2
  Vdc : Inport  Port=3
  Ia : Inport  Port=4
  Ib : Inport  Port=5
  PhaseShortEnableFlag : Inport  Port=6
  getDutyandSample : Subsystem
  invClarkeTransform : Subsystem
  DutySVPWM : Outport
  SamplePoint : Outport  Port=2
  SectorN : Outport  Port=3
  wires:
  getDutyandSample/2(SamplePoint) -> SamplePoint/1
  getDutyandSample/1(DutyABC) -> DutySVPWM/1
  Ib/1 -> getDutyandSample/5(ib)
  Ia/1 -> getDutyandSample/4(Ia)
  getDutyandSample/3(SectorN) -> SectorN/1
  PhaseShortEnableFlag/1 -> getDutyandSample/6(PhaseShortEnableFlag)
  invClarkeTransform/1(Va) -> getDutyandSample/1(Va)
  invClarkeTransform/2(Vb) -> getDutyandSample/2(Vb)
  invClarkeTransform/3(Vc) -> getDutyandSample/3(Vc)
  Valpha/1 -> invClarkeTransform/1(Valpha)
  Vbeta/1 -> invClarkeTransform/2(Vbeta)
  Vdc/1 -> invClarkeTransform/3(Vdc)

== system WiperCtrl/HighFrequency/voltageLimit ==
  UdRef : Inport
  UqRef : Inport  Port=2
  Umax : Inport  Port=3
  Constant : Constant
  Constant1 : Constant
  Terminator : Terminator
  Terminator1 : Terminator
  Terminator2 : Terminator
  Ud : Outport
  Uq : Outport  Port=2
  wires:
  UdRef/1 -> Terminator/1
  Constant/1 -> Ud/1
  Constant1/1 -> Uq/1
  UqRef/1 -> Terminator1/1
  Umax/1 -> Terminator2/1

== system WiperCtrl/Hardware_Math/CurrentSample/CurrentSample(OneRS)  ==
  SampleTrigger : Inport
  Current : Inport  Port=2
  CurrentSample1 : Subsystem  TreatAsAtomicUnit=on
  CurrentSample2 : Subsystem  Variant=on  VariantControlMode=label  VariantControl=CurrentSample2  LabelModeActiveChoice=CurrentSample2
  Demux : Demux  Outputs=2
  Mux : Mux  Inputs=2
  CurrentSample : Outport
  wires:
  CurrentSample2/1(CurrentSample2) -> Mux/2
  Demux/2 -> CurrentSample2/Trigger
  Current/1 -> CurrentSample2/1(Current), CurrentSample1/1(Current)
  Mux/1 -> CurrentSample/1
  CurrentSample1/1(CurrentSample1) -> Mux/1
  SampleTrigger/1 -> Demux/1
  Demux/1 -> CurrentSample1/Trigger

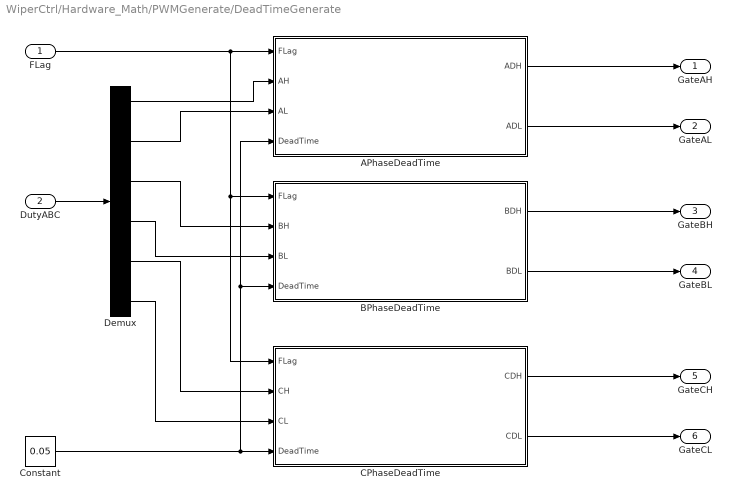
== system WiperCtrl/Hardware_Math/PWMGenerate/DeadTimeGenerate ==
  FLag : Inport
  DutyABC : Inport  Port=2
  APhaseDeadTime : Subsystem
  BPhaseDeadTime : Subsystem
  CPhaseDeadTime : Subsystem
  Constant : Constant  Value=0.05  SampleTime=-1
  Demux : Demux  Outputs=6
  GateAH : Outport
  GateAL : Outport  Port=2
  GateBH : Outport  Port=3
  GateBL : Outport  Port=4
  GateCH : Outport  Port=5
  GateCL : Outport  Port=6
  wires:
  Demux/6 -> CPhaseDeadTime/3(CL)
  Demux/5 -> CPhaseDeadTime/2(CH)
  Demux/4 -> BPhaseDeadTime/3(BL)
  Demux/3 -> BPhaseDeadTime/2(BH)
  Demux/2 -> APhaseDeadTime/3(AL)
  Demux/1 -> APhaseDeadTime/2(AH)
  DutyABC/1 -> Demux/1
  CPhaseDeadTime/1(CDH) -> GateCH/1
  CPhaseDeadTime/2(CDL) -> GateCL/1
  BPhaseDeadTime/1(BDH) -> GateBH/1
  BPhaseDeadTime/2(BDL) -> GateBL/1
  APhaseDeadTime/2(ADL) -> GateAL/1
  FLag/1 -> CPhaseDeadTime/1(FLag), BPhaseDeadTime/1(FLag), APhaseDeadTime/1(FLag)
  Constant/1 -> APhaseDeadTime/4(DeadTime), BPhaseDeadTime/4(DeadTime), CPhaseDeadTime/4(DeadTime)
  APhaseDeadTime/1(ADH) -> GateAH/1

== system WiperCtrl/HighFrequency/currentReconstruction/currentPreProcess ==
  SampleCurrentPoint1 : Inport
  SampleCurrentPoint2 : Inport  Port=2
  Gain : Gain  Gain=-1
  Subtract : Sum  Inputs=--
  I1 : Outport
  -I2 : Outport  Port=2
  I2-I1 : Outport  Port=3
  wires:
  SampleCurrentPoint2/1 -> Gain/1
  SampleCurrentPoint1/1 -> I1/1, Subtract/1  "I1"
  Subtract/1 -> I2-I1/1  "I2-I1"
  Gain/1 -> -I2/1, Subtract/2  "-I2"

== system WiperCtrl/HighFrequency/currentReconstruction/getCurrentPhase ==
  SectorN : Inport
  I1 : Inport  Port=2
  -I2 : Inport  Port=3
  I2-I1 : Inport  Port=4
  getCurrentPhaseA : Subsystem
  getCurrentPhaseB : Subsystem
  Ia : Outport
  Ib : Outport  Port=2
  wires:
  SectorN/1 -> getCurrentPhaseB/1(SectorN), getCurrentPhaseA/1(SectorN)
  I1/1 -> getCurrentPhaseB/2(I1), getCurrentPhaseA/2(I1)
  -I2/1 -> getCurrentPhaseB/3(-I2), getCurrentPhaseA/3(-I2)
  I2-I1/1 -> getCurrentPhaseB/4(I2-I1), getCurrentPhaseA/4(I2-I1)
  getCurrentPhaseA/1(Ia) -> Ia/1
  getCurrentPhaseB/1(Ib) -> Ib/1

== system WiperCtrl/HighFrequency/observation/flux ==
  Ualpha : Inport
  Ubeta : Inport  Port=2
  Ialpha : Inport  Port=3
  Ibeta : Inport  Port=4
  Constant : Constant
  Terminator{,1..3} (4 alike) : Terminator
  Speed : Outport
  Theta : Outport  Port=2
  wires:
  Ibeta/1 -> Terminator3/1
  Constant/1 -> Speed/1, Theta/1
  Ubeta/1 -> Terminator1/1
  Ualpha/1 -> Terminator/1
  Ialpha/1 -> Terminator2/1

== system WiperCtrl/HighFrequency/observation/longbergur ==
  Ualpha : Inport
  Ubeta : Inport  Port=2
  Ialpha : Inport  Port=3
  Ibeta : Inport  Port=4
  Constant : Constant
  Terminator{,1..3} (4 alike) : Terminator
  Speed : Outport
  Theta : Outport  Port=2
  wires:
  Ibeta/1 -> Terminator3/1
  Constant/1 -> Speed/1, Theta/1
  Ubeta/1 -> Terminator1/1
  Ualpha/1 -> Terminator/1
  Ialpha/1 -> Terminator2/1

== system WiperCtrl/HighFrequency/observation/smo ==
  Ualpha : Inport
  Ubeta : Inport  Port=2
  Ialpha : Inport  Port=3
  Ibeta : Inport  Port=4
  Constant : Constant
  Terminator{,1..3} (4 alike) : Terminator
  Speed : Outport
  Theta : Outport  Port=2
  wires:
  Ualpha/1 -> Terminator/1
  Ubeta/1 -> Terminator1/1
  Ibeta/1 -> Terminator3/1
  Ialpha/1 -> Terminator2/1
  Constant/1 -> Speed/1, Theta/1

== system WiperCtrl/HighFrequency/pidForCurrentD/pidConcatenation ==
  Ref : Inport
  Real : Inport  Port=2
  Add : Sum
  Add1 : Sum
  Delay One Step : Delay  DelayLength=1
  Gain : Gain
  Gain1 : Gain
  Saturation : Saturate
  Saturation1 : Saturate
  Subtract : Sum  Inputs=+-
  PIOut : Outport
  wires:
  Ref/1 -> Subtract/1
  Saturation1/1 -> PIOut/1
  Saturation/1 -> Add1/2
  Add1/1 -> Saturation1/1
  Gain1/1 -> Add/1
  Subtract/1 -> Gain/1
  Add/1 -> Delay One Step/1, Saturation/1
  Real/1 -> Subtract/2
  Delay One Step/1 -> Add/2
  Gain/1 -> Add1/1, Gain1/1

== system WiperCtrl/HighFrequency/pidForCurrentD/pidPallarConnection ==
  Ref : Inport
  Real : Inport  Port=2
  Add : Sum
  Add1 : Sum
  Delay One Step : Delay  DelayLength=1
  Gain : Gain
  Gain1 : Gain
  Saturation : Saturate
  Saturation1 : Saturate
  Subtract : Sum  Inputs=+-
  PIOut : Outport
  wires:
  Delay One Step/1 -> Add/2
  Real/1 -> Subtract/2
  Gain/1 -> Add1/1
  Add/1 -> Delay One Step/1, Saturation/1
  Subtract/1 -> Gain1/1, Gain/1
  Gain1/1 -> Add/1
  Add1/1 -> Saturation1/1
  Saturation/1 -> Add1/2
  Saturation1/1 -> PIOut/1
  Ref/1 -> Subtract/1

== system WiperCtrl/HighFrequency/pidForCurrentQ/pidConcatenation ==
  Ref : Inport
  Real : Inport  Port=2
  Add : Sum
  Add1 : Sum
  Delay One Step : Delay  DelayLength=1
  Gain : Gain
  Gain1 : Gain
  Saturation : Saturate
  Saturation1 : Saturate
  Subtract : Sum  Inputs=+-
  PIOut : Outport
  wires:
  Gain/1 -> Gain1/1, Add1/1
  Delay One Step/1 -> Add/2
  Real/1 -> Subtract/2
  Add/1 -> Saturation/1, Delay One Step/1
  Subtract/1 -> Gain/1
  Gain1/1 -> Add/1
  Add1/1 -> Saturation1/1
  Saturation/1 -> Add1/2
  Saturation1/1 -> PIOut/1
  Ref/1 -> Subtract/1

== system WiperCtrl/HighFrequency/pidForCurrentQ/pidPallarConnection ==
  Ref : Inport
  Real : Inport  Port=2
  Add : Sum
  Add1 : Sum
  Delay One Step : Delay  DelayLength=1
  Gain : Gain
  Gain1 : Gain
  Saturation : Saturate
  Saturation1 : Saturate
  Subtract : Sum  Inputs=+-
  PIOut : Outport
  wires:
  Ref/1 -> Subtract/1
  Saturation1/1 -> PIOut/1
  Saturation/1 -> Add1/2
  Add1/1 -> Saturation1/1
  Gain1/1 -> Add/1
  Subtract/1 -> Gain/1, Gain1/1
  Add/1 -> Delay One Step/1, Saturation/1
  Gain/1 -> Add1/1
  Real/1 -> Subtract/2
  Delay One Step/1 -> Add/2

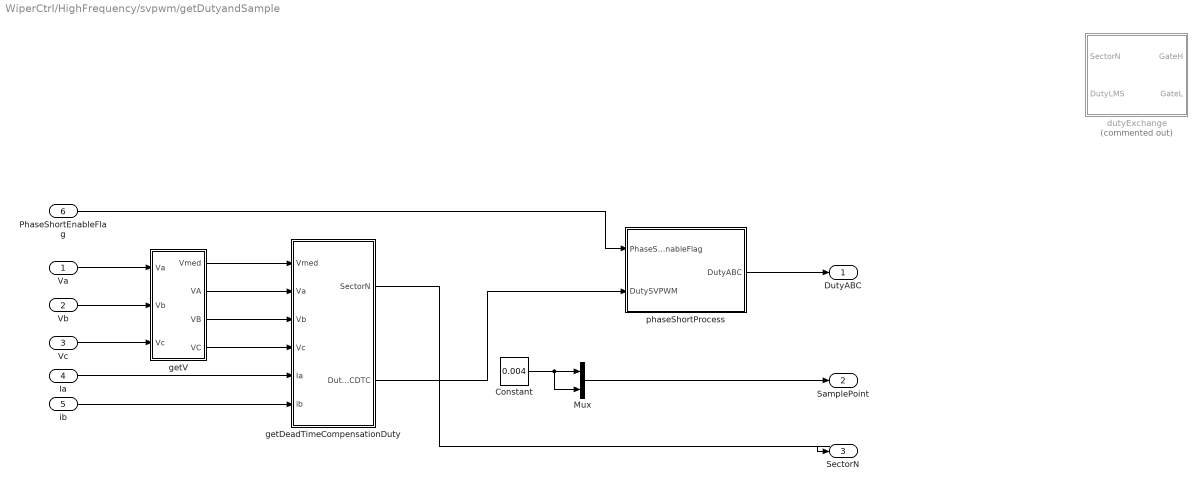
== system WiperCtrl/HighFrequency/svpwm/getDutyandSample ==
  Va : Inport
  Vb : Inport  Port=2
  Vc : Inport  Port=3
  Ia : Inport  Port=4
  ib : Inport  Port=5
  PhaseShortEnableFlag : Inport  Port=6
  Constant : Constant  Value=0.004
  Mux : Mux  Inputs=2
  dutyExchange : Subsystem  Commented=on
  getDeadTimeCompensationDuty : Subsystem
  getV : Subsystem
  phaseShortProcess : Subsystem
  DutyABC : Outport
  SamplePoint : Outport  Port=2
  SectorN : Outport  Port=3
  wires:
  Va/1 -> getV/1(Va)
  Vb/1 -> getV/2(Vb)
  Vc/1 -> getV/3(Vc)
  getV/1(Vmed) -> getDeadTimeCompensationDuty/1(Vmed)
  Ia/1 -> getDeadTimeCompensationDuty/5(Ia)
  ib/1 -> getDeadTimeCompensationDuty/6(ib)
  getV/2(VA) -> getDeadTimeCompensationDuty/2(Va)
  getV/3(VB) -> getDeadTimeCompensationDuty/3(Vb)
  getV/4(VC) -> getDeadTimeCompensationDuty/4(Vc)
  getDeadTimeCompensationDuty/1(SectorN) -> SectorN/1
  Mux/1 -> SamplePoint/1
  phaseShortProcess/1(DutyABC) -> DutyABC/1
  PhaseShortEnableFlag/1 -> phaseShortProcess/1(PhaseShortEnableFlag)
  getDeadTimeCompensationDuty/2(DutyABCDTC) -> phaseShortProcess/2(DutySVPWM)
  Constant/1 -> Mux/2, Mux/1

== system WiperCtrl/HighFrequency/svpwm/invClarkeTransform ==
  Valpha : Inport
  Vbeta : Inport  Port=2
  Vdc : Inport  Port=3
  Divide : Product  Inputs=*/
  Divide1 : Product  Inputs=*/
  getSectorN : Subsystem  Commented=on
  invClarkeTransform : Subsystem
  Va : Outport
  Vb : Outport  Port=2
  Vc : Outport  Port=3
  wires:
  Divide/1 -> invClarkeTransform/1(Valpha)
  Divide1/1 -> invClarkeTransform/2(Vbeta)
  invClarkeTransform/1(Va) -> Va/1
  invClarkeTransform/3(Vc) -> Vc/1
  invClarkeTransform/2(Vb) -> Vb/1
  Valpha/1 -> Divide/1
  Vbeta/1 -> Divide1/1
  Vdc/1 -> Divide/2, Divide1/2

== system WiperCtrl/Hardware_Math/CurrentSample/CurrentSample(OneRS) /CurrentSample1 ==
  Current : Inport
  Trigger : TriggerPort  VariantControl=(inherit)  InitialTriggerSignalState=zero
  ADCOffset : Constant  Value=0  SampleTime=-1
  ADCQuality : Gain  Gain=1024/5
  Add : Sum
  CSAGain : Gain  Gain=50
  CurrentSample1 : Outport
  wires:
  Current/1 -> CSAGain/1
  CSAGain/1 -> Add/2
  ADCOffset/1 -> Add/1
  Add/1 -> ADCQuality/1
  ADCQuality/1 -> CurrentSample1/1

== system WiperCtrl/Hardware_Math/CurrentSample/CurrentSample(OneRS) /CurrentSample2 ==
  Current : Inport
  Trigger : TriggerPort  TriggerType=either  VariantControl=(inherit)
  CurrentSample2Down : Subsystem  TreatAsAtomicUnit=on  VariantControl=CurrentSample2
  CurrentSample2Up : Subsystem  TreatAsAtomicUnit=on  VariantControl=CurrentSample2 1
  CurrentSample2 : Outport

== system WiperCtrl/Hardware_Math/PWMGenerate/DeadTimeGenerate/APhaseDeadTime ==
  FLag : Inport
  AH : Inport  Port=2
  AL : Inport  Port=3
  DeadTime : Inport  Port=4
  Add : Sum
  Subtract : Sum  Inputs=+-
  Switch : Switch  Criteria=u2 > Threshold  SaturateOnIntegerOverflow=off  InputSameDT=off
  Switch1 : Switch  Criteria=u2 > Threshold  SaturateOnIntegerOverflow=off  InputSameDT=off
  ADH : Outport
  ADL : Outport  Port=2
  wires:
  DeadTime/1 -> Add/2, Subtract/2
  AL/1 -> Subtract/1
  FLag/1 -> Switch/2, Switch1/2
  Add/1 -> Switch/1
  Switch/1 -> ADH/1  "ADH"
  AH/1 -> Switch1/1, Switch/3, Add/1
  Subtract/1 -> Switch1/3
  Switch1/1 -> ADL/1  "ADL"

== system WiperCtrl/Hardware_Math/PWMGenerate/DeadTimeGenerate/BPhaseDeadTime ==
  FLag : Inport
  BH : Inport  Port=2
  BL : Inport  Port=3
  DeadTime : Inport  Port=4
  Add : Sum
  Subtract : Sum  Inputs=+-
  Switch : Switch  Criteria=u2 > Threshold  SaturateOnIntegerOverflow=off  InputSameDT=off
  Switch1 : Switch  Criteria=u2 > Threshold  SaturateOnIntegerOverflow=off  InputSameDT=off
  BDH : Outport
  BDL : Outport  Port=2
  wires:
  Switch1/1 -> BDL/1  "BDL"
  Subtract/1 -> Switch1/3
  BH/1 -> Add/1, Switch/3, Switch1/1
  Switch/1 -> BDH/1  "BDH"
  Add/1 -> Switch/1
  FLag/1 -> Switch1/2, Switch/2
  BL/1 -> Subtract/1
  DeadTime/1 -> Subtract/2, Add/2

== system WiperCtrl/Hardware_Math/PWMGenerate/DeadTimeGenerate/CPhaseDeadTime ==
  FLag : Inport
  CH : Inport  Port=2
  CL : Inport  Port=3
  DeadTime : Inport  Port=4
  Add : Sum
  Subtract : Sum  Inputs=+-
  Switch : Switch  Criteria=u2 > Threshold  SaturateOnIntegerOverflow=off  InputSameDT=off
  Switch1 : Switch  Criteria=u2 > Threshold  SaturateOnIntegerOverflow=off  InputSameDT=off
  CDH : Outport
  CDL : Outport  Port=2
  wires:
  DeadTime/1 -> Add/2, Subtract/2
  CL/1 -> Subtract/1
  FLag/1 -> Switch/2, Switch1/2
  Add/1 -> Switch/1
  Switch/1 -> CDH/1  "CDH"
  CH/1 -> Switch1/1, Switch/3, Add/1
  Subtract/1 -> Switch1/3
  Switch1/1 -> CDL/1  "CDL"

== system WiperCtrl/HighFrequency/currentReconstruction/getCurrentPhase/getCurrentPhaseA ==
  note: Sector = 7 => A>B>C
      | Sector = 6 => A>C>B
      | Sector = 3 => B>A>C
      | Sector = 1 => B>C>A
      | Sector = 4 => C>A>B
      | Sector = 0 => C>B>A
  SectorN : Inport
  I1 : Inport  Port=2
  -I2 : Inport  Port=3
  I2-I1 : Inport  Port=4
  Delay One Step : Delay  DelayLength=1
  Multiport Switch : MultiPortSwitch  DataPortOrder=Specify indices  Inputs=8  DataPortIndices={0,1,3,4,6,7}  DataPortForDefault=Additional data port  SaturateOnIntegerOverflow=off  InputSameDT=off
  Ia : Outport
  wires:
  SectorN/1 -> Multiport Switch/1
  Multiport Switch/1 -> Ia/1, Delay One Step/1  "Ia"
  -I2/1 -> Multiport Switch/3, Multiport Switch/2
  I1/1 -> Multiport Switch/7, Multiport Switch/6
  I2-I1/1 -> Multiport Switch/5, Multiport Switch/4
  Delay One Step/1 -> Multiport Switch/8  "Ia_Last"

== system WiperCtrl/HighFrequency/currentReconstruction/getCurrentPhase/getCurrentPhaseB ==
  note: Sector = 7 => A>B>C
      | Sector = 6 => A>C>B
      | Sector = 3 => B>A>C
      | Sector = 1 => B>C>A
      | Sector = 4 => C>A>B
      | Sector = 0 => C>B>A
  SectorN : Inport
  I1 : Inport  Port=2
  -I2 : Inport  Port=3
  I2-I1 : Inport  Port=4
  Delay One Step : Delay  DelayLength=1
  Multiport Switch : MultiPortSwitch  DataPortOrder=Specify indices  Inputs=8  DataPortIndices={0,1,3,4,6,7}  DataPortForDefault=Additional data port  SaturateOnIntegerOverflow=off  InputSameDT=off
  Ib : Outport
  wires:
  Multiport Switch/1 -> Ib/1, Delay One Step/1  "Ib"
  SectorN/1 -> Multiport Switch/1
  I1/1 -> Multiport Switch/4, Multiport Switch/3
  I2-I1/1 -> Multiport Switch/7, Multiport Switch/2
  -I2/1 -> Multiport Switch/6, Multiport Switch/5
  Delay One Step/1 -> Multiport Switch/8  "Ib_Last"

== system WiperCtrl/HighFrequency/svpwm/getDutyandSample/dutyExchange ==
  SectorN : Inport
  DutyLMS : Inport  Port=2
  Demux : Demux  Outputs=6
  gateHtoPhase : Subsystem
  gateLtoPhase : Subsystem
  GateH : Outport
  GateL : Outport  Port=2
  wires:
  DutyLMS/1 -> Demux/1
  Demux/1 -> gateHtoPhase/2(DutyLH)  "DU\\utyLH"
  Demux/2 -> gateLtoPhase/2(DutyLH)  "DutyLL"
  Demux/3 -> gateHtoPhase/3(DutyMH)  "DutyMH"
  Demux/4 -> gateLtoPhase/3(DutyMH)  "DutyML"
  Demux/5 -> gateHtoPhase/4(DutySH)  "DutySH"
  Demux/6 -> gateLtoPhase/4(DutySH)  "DutySL"
  gateHtoPhase/1(GateH) -> GateH/1
  gateLtoPhase/1(GateL) -> GateL/1
  SectorN/1 -> gateLtoPhase/1(SectorN), gateHtoPhase/1(SectorN)

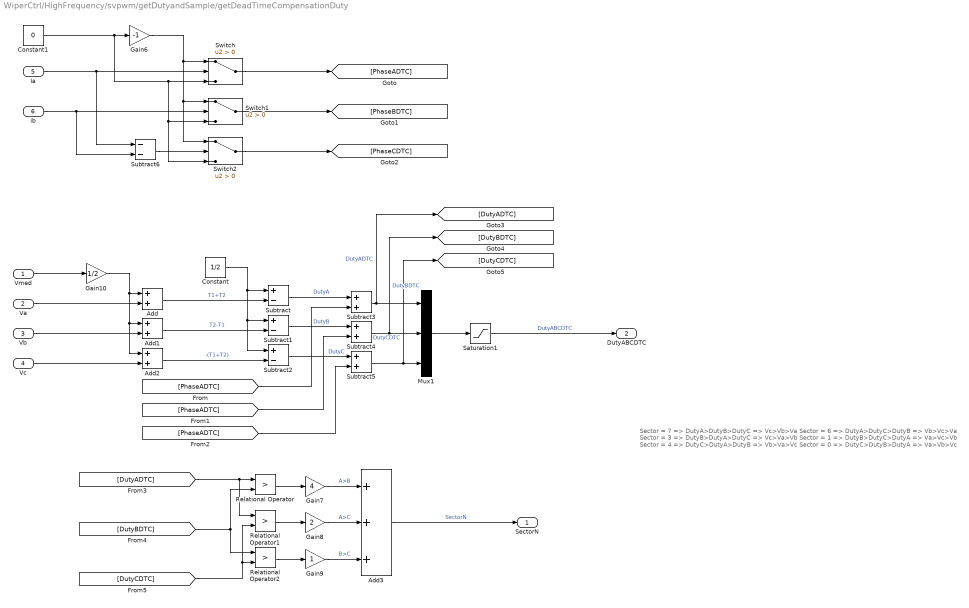
== system WiperCtrl/HighFrequency/svpwm/getDutyandSample/getDeadTimeCompensationDuty ==
  note: Sector = 7 => DutyA>DutyB>DutyC => Vc>Vb>Va
      | Sector = 6 => DutyA>DutyC>DutyB => Vb>Vc>Va
      | Sector = 3 => DutyB>DutyA>DutyC => Vc>Va>Vb
      | Sector = 1 => DutyB>DutyC>DutyA => Va>Vc>Vb
      | Sector = 4 => DutyC>DutyA>DutyB => Vb>Va>Vc
      | Sector = 0 => DutyC>DutyB>DutyA => Va>Vb>Vc
  Vmed : Inport
  Va : Inport  Port=2
  Vb : Inport  Port=3
  Vc : Inport  Port=4
  Ia : Inport  Port=5
  ib : Inport  Port=6
  Add : Sum
  Add1 : Sum
  Add2 : Sum
  Add3 : Sum  Inputs=+++
  Constant : Constant  Value=1/2  SampleTime=MC_Sim_HighFrequenceStep
  Constant1 : Constant  Value=0
  Gain10 : Gain  Gain=1/2
  Gain6 : Gain  Gain=-1
  Gain7 : Gain  Gain=4
  Gain8 : Gain  Gain=2
  Gain9 : Gain
  Mux1 : Mux  Inputs=3
  Relational Operator : RelationalOperator  Operator=>  OutDataTypeStr=boolean  RndMeth=Simplest  InputSameDT=off
  Relational Operator1 : RelationalOperator  Operator=>  OutDataTypeStr=boolean  RndMeth=Simplest  InputSameDT=off
  Relational Operator2 : RelationalOperator  Operator=>  OutDataTypeStr=boolean  RndMeth=Simplest  InputSameDT=off
  Saturation1 : Saturate  UpperLimit=MC_SVPWM_DutyMax  LowerLimit=MC_SVPWM_DutyMin
  Subtract : Sum  Inputs=+-
  Subtract1 : Sum  Inputs=+-
  Subtract2 : Sum  Inputs=+-
  Subtract3 : Sum
  Subtract4 : Sum
  Subtract5 : Sum
  Subtract6 : Sum  Inputs=--
  Switch : Switch  Criteria=u2 > Threshold  SaturateOnIntegerOverflow=off  InputSameDT=off
  Switch1 : Switch  Criteria=u2 > Threshold  SaturateOnIntegerOverflow=off  InputSameDT=off
  Switch2 : Switch  Criteria=u2 > Threshold  SaturateOnIntegerOverflow=off  InputSameDT=off
  SectorN : Outport
  DutyABCDTC : Outport  Port=2
  wires:
  Va/1 -> Add/2
  Vmed/1 -> Gain10/1
  Vb/1 -> Add1/2
  Vc/1 -> Add2/2
  Add/1 -> Subtract/2  "T1+T2"
  Add2/1 -> Subtract2/2  "-(T1+T2)"
  Add1/1 -> Subtract1/2  "T2-T1"
  Constant/1 -> Subtract2/1, Subtract1/1, Subtract/1
  Subtract/1 -> Subtract3/1  "DutyA"
  Subtract1/1 -> Subtract4/1  "DutyB"
  Subtract2/1 -> Subtract5/1  "DutyC"
  Subtract3/1 -> [DutyADTC], Mux1/1  "DutyADTC"
  Subtract4/1 -> [DutyBDTC], Mux1/2  "DutyBDTC"
  Subtract5/1 -> [DutyCDTC], Mux1/3  "DutyCDTC"
  Mux1/1 -> Saturation1/1
  Saturation1/1 -> DutyABCDTC/1  "DutyABCDTC"
  Ia/1 -> Subtract6/1, Switch/2
  Gain6/1 -> Switch2/1, Switch1/1, Switch/1
  ib/1 -> Subtract6/2, Switch1/2
  Subtract6/1 -> Switch2/2
  Constant1/1 -> Switch2/3, Switch1/3, Switch/3, Gain6/1
  Switch/1 -> [PhaseADTC]
  Switch1/1 -> [PhaseBDTC]
  Switch2/1 -> [PhaseCDTC]
  [PhaseADTC] -> Subtract3/2
  [PhaseADTC] -> Subtract4/2
  [PhaseADTC] -> Subtract5/2
  [DutyBDTC] -> Relational Operator2/1, Relational Operator/2
  [DutyADTC] -> Relational Operator1/1, Relational Operator/1
  [DutyCDTC] -> Relational Operator2/2, Relational Operator1/2
  Relational Operator/1 -> Gain7/1
  Relational Operator1/1 -> Gain8/1
  Relational Operator2/1 -> Gain9/1
  Gain8/1 -> Add3/2  "A>C"
  Gain9/1 -> Add3/3  "B>C"
  Gain7/1 -> Add3/1  "A>B"
  Add3/1 -> SectorN/1  "SectorN"
  Gain10/1 -> Add2/1, Add1/1, Add/1

== system WiperCtrl/HighFrequency/svpwm/getDutyandSample/getV ==
  Va : Inport
  Vb : Inport  Port=2
  Vc : Inport  Port=3
  Add : Sum
  Gain : Gain  Gain=-1
  getVmax : Subsystem
  getVmin : Subsystem
  Vmed : Outport
  VA : Outport  Port=2
  VB : Outport  Port=3
  VC : Outport  Port=4
  wires:
  Gain/1 -> Vmed/1  "Vmed"
  getVmin/1(Vmin) -> Add/2
  Va/1 -> VA/1, getVmin/1(Va), getVmax/1(Va)
  getVmax/1(Vmax) -> Add/1
  Add/1 -> Gain/1
  Vb/1 -> getVmin/2(Vb), VB/1, getVmax/2(Vb)
  Vc/1 -> VC/1, getVmin/3(Vc), getVmax/3(Vc)

== system WiperCtrl/HighFrequency/svpwm/getDutyandSample/phaseShortProcess ==
  PhaseShortEnableFlag : Inport
  DutySVPWM : Inport  Port=2
  Constant : Constant  Value=0
  Demux : Demux  Outputs=3
  Mux : Mux  Inputs=6
  Mux1 : Mux  Inputs=6
  Switch : Switch  Criteria=u2 > Threshold  SaturateOnIntegerOverflow=off  InputSameDT=off
  DutyABC : Outport
  wires:
  PhaseShortEnableFlag/1 -> Switch/2
  Constant/1 -> Mux/6, Mux/5, Mux/4, Mux/3, Mux/2, Mux/1
  Mux/1 -> Switch/1
  Switch/1 -> DutyABC/1  "DutyABC[6]"
  DutySVPWM/1 -> Demux/1
  Demux/1 -> Mux1/2, Mux1/1
  Demux/2 -> Mux1/4, Mux1/3
  Demux/3 -> Mux1/6, Mux1/5
  Mux1/1 -> Switch/3

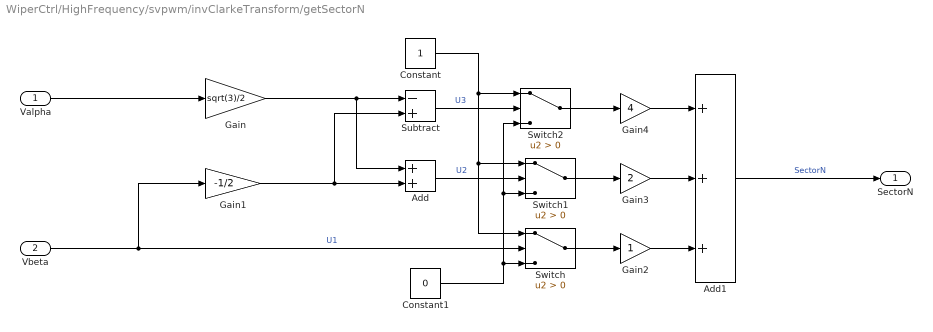
== system WiperCtrl/HighFrequency/svpwm/invClarkeTransform/getSectorN ==
  Valpha : Inport
  Vbeta : Inport  Port=2
  Add : Sum
  Add1 : Sum  Inputs=+++
  Constant : Constant
  Constant1 : Constant  Value=0
  Gain : Gain  Gain=sqrt(3)/2
  Gain1 : Gain  Gain=-1/2
  Gain2 : Gain
  Gain3 : Gain  Gain=2
  Gain4 : Gain  Gain=4
  Subtract : Sum  Inputs=-+
  Switch : Switch  Criteria=u2 > Threshold  SaturateOnIntegerOverflow=off  InputSameDT=off
  Switch1 : Switch  Criteria=u2 > Threshold  SaturateOnIntegerOverflow=off  InputSameDT=off
  Switch2 : Switch  Criteria=u2 > Threshold  SaturateOnIntegerOverflow=off  InputSameDT=off
  SectorN : Outport
  wires:
  Constant/1 -> Switch1/1, Switch/1, Switch2/1
  Gain3/1 -> Add1/2
  Gain1/1 -> Add/2, Subtract/2
  Switch/1 -> Gain2/1
  Gain/1 -> Add/1, Subtract/1
  Switch1/1 -> Gain3/1
  Vbeta/1 -> Switch/2, Gain1/1  "U1"
  Constant1/1 -> Switch2/3, Switch1/3, Switch/3
  Valpha/1 -> Gain/1
  Subtract/1 -> Switch2/2  "U3"
  Gain2/1 -> Add1/3
  Switch2/1 -> Gain4/1
  Add/1 -> Switch1/2  "U2"
  Gain4/1 -> Add1/1
  Add1/1 -> SectorN/1  "SectorN"
